simulink model "Buck_Converter_with_3ph_Full_Bridge_Rectifier_v2"  (R2022b)
settings: Solver=VariableStepAuto  StartTime=0.0  StopTime=3  RelTol=1e-3
libraries: spsDiodeLib x7, spsRMSLib x4, spsCurrentMeasurementLib x3, spsSeriesRLCBranchLib x3, spsVoltageMeasurementLib x2, slpidlib x1, simulink x1, spsDCMachineLib x1, spsDCVoltageSourceLib x1, spsGroundLib x1, spsIGBTDiodeLib x1, spsPower3phInstantaneousLib x1
settings Model: Creator=meteh  LastModifiedBy=meteh
settings SolverCC: ZeroCrossAlgorithm=Adaptive
settings DebuggingCC: IgnoredZcDiagnostic=none

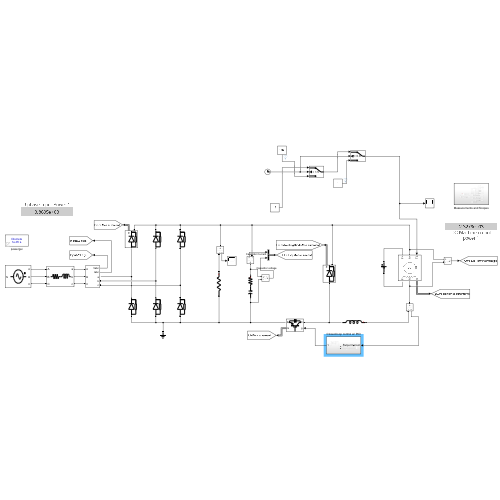
[thumbnail: Simulink's stored preview of the top-level diagram]
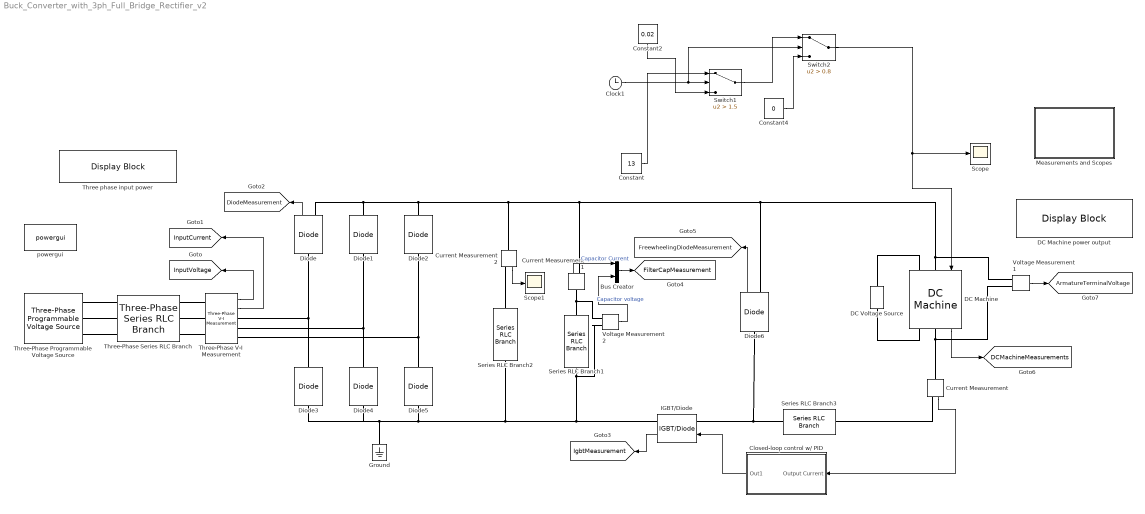
== system Buck_Converter_with_3ph_Full_Bridge_Rectifier_v2 ==
  Bus Creator : BusCreator  Inputs=2
  Clock1 : Clock
  Closed-loop control w/ PID : Subsystem
  Constant : Constant  Value=13
  Constant2 : Constant  Value=0.02
  Constant4 : Constant  Value=0
  Current Measurement : spsCurrentMeasurementLib/Current Measurement  PhasorSimulation=off  OutputType=Complex  PSBequivalent=0
  Current Measurement1 : spsCurrentMeasurementLib/Current Measurement  PhasorSimulation=off  OutputType=Complex  PSBequivalent=0
  Current Measurement2 : spsCurrentMeasurementLib/Current Measurement  PhasorSimulation=off  OutputType=Complex  PSBequivalent=0
  DC Machine : spsDCMachineLib/DC Machine  PresetModel=No  MechanicalLoad=Torque TL  FieldType=Wound  ShowDetailedParameters=on  MeasurementBus=off  RLa="[ 0.8  0.0125]"  RLf="[ 210  23]"  Laf=1  MachineConstant=Torque constant (N.m/A)  Ke=1.8  Kt=1.8  J=0.001  Bm=0.001  Tf=0.001  w0=0  Ifinit=0  TsPowergui=0  TsBlock=-1
  DC Machine power output : DisplayBlock  LabelPosition=Bottom  Transparency=1
  DC Voltage Source : spsDCVoltageSourceLib/DC Voltage Source  Amplitude=200  Measurements=None
  Diode : spsDiodeLib/Diode  Ron=0.001  Lon=0  Vf=0.8  IC=0  UseSnubber=0  Rs=500  Cs=250e-9  Measurements=on
  Diode{1..5} (5 alike) : spsDiodeLib/Diode  Ron=0.001  Lon=0  Vf=0.8  IC=0  UseSnubber=0  Rs=500  Cs=250e-9  Measurements=off
  Diode6 : spsDiodeLib/Diode  Ron=0.001  Lon=0  Vf=0.8  IC=0  UseSnubber=0  Rs=120  Cs=250e-9  Measurements=on
  Ground : spsGroundLib/Ground  LConnTagsString=a
  IGBT/Diode : spsIGBTDiodeLib/IGBT//Diode  Ron=1e-2  Rs=120  Cs=250e-9  Measurements=on
  Measurements and Scopes : Subsystem
  Scope : Scope
  Scope1 : Scope
  Series RLC Branch1 : spsSeriesRLCBranchLib/Series RLC Branch  LConnTagsString=__new0  RConnTagsString=__new0  BranchType=RC  Resistance=0.01  Inductance=12.5e-3  SetiL0=off  InitialCurrent=0  Capacitance=940e-6  Setx0=off  InitialVoltage=0  Measurements=None
  Series RLC Branch2 : spsSeriesRLCBranchLib/Series RLC Branch  LConnTagsString=__new0  RConnTagsString=__new0  BranchType=R  Resistance=5.6e3  Inductance=12.5e-3  SetiL0=off  InitialCurrent=0  Capacitance=940e-6  Setx0=off  InitialVoltage=0  Measurements=None
  Series RLC Branch3 : spsSeriesRLCBranchLib/Series RLC Branch  LConnTagsString=__new0  RConnTagsString=__new0  BranchType=L  Resistance=0.01  Inductance=10e-9  SetiL0=off  InitialCurrent=0  Capacitance=940e-6  Setx0=off  InitialVoltage=0  Measurements=None
  Switch1 : Switch  Criteria=u2 > Threshold  Threshold=1.5  SaturateOnIntegerOverflow=off  InputSameDT=off
  Switch2 : Switch  Criteria=u2 > Threshold  Threshold=0.8  SaturateOnIntegerOverflow=off  InputSameDT=off
  Three phase input power : DisplayBlock  Description=Three phase input power  Transparency=1  Layout=Fill available space
  Three-Phase Programmable Voltage Source : spsThreePhaseProgrammableVoltageSourceLib/Three-Phase Programmable Voltage Source  PositiveSequence="[133  0 50]"  VariationEntity=Amplitude  VariationType=Table of time-amplitude pairs  VariationTypeAlt=Step  VariationStep=0.5  VariationRate=10  VariationMagnitude=0.3  VariationFrequency=2  VariationTiming=[1 2]  VariationPhaseA=off  Amplitudes=[0 0.25 0.5 0.75 1.0]  TimeValues=[0 0.2 0.4 0.6 0.8]  HarmonicGeneration=off  HarmonicA=[3 0.2 -25 0]  HarmonicB=[2 0.15 35 2]  Timing="[0.05  3]"  BusType=swing  Pref=0  Qref=0  Qmin=-inf  Qmax=inf
  Three-Phase Series RLC Branch : spsThreePhaseSeriesRLCBranchLib/Three-Phase Series RLC Branch  LConnTagsString=A|B|C  RConnTagsString=A|B|C  BranchType=RL  Resistance=1e-3  Inductance=2e-3  Capacitance=1e-6  Measurements=None
  Three-Phase V-I Measurement : spsThreePhaseVIMeasurementLib/Three-Phase V-I Measurement  VoltageMeasurement=phase-to-ground  SetLabelV=off  LabelV=Vabc  Vpu=off  VpuLL=off  CurrentMeasurement=yes  SetLabelI=off  LabelI=Iabc  Ipu=off  Pbase=100e6  Vbase=500e3  OutputType=Complex  PhasorSimulation=off  PSBequivalent=0
  Voltage Measurement1 : spsVoltageMeasurementLib/Voltage Measurement  PhasorSimulation=off  OutputType=Complex  PSBequivalent=0
  Voltage Measurement2 : spsVoltageMeasurementLib/Voltage Measurement  PhasorSimulation=off  OutputType=Complex  PSBequivalent=0
  powergui : spspowerguiLib/powergui  Priority=1  SimulationMode=Discrete  SampleTime=1e-5  frequency=60  Iterations=50  frequencyindice=0  Pbase=100e6  ErrMax=1e-4  UnitsV=kV  UnitsW=MW  buscounter=0  FunctionMessages=off  echomessages=off  EnableUseOfTLC=off  CurrentSourceSwitches=on  DisableSnubberDevices=off  DisableRonSwitches=off  DisableVfSwitches=off  DisplayEquations=off  AutomaticDiscreteSolvers=off  SolverType=Tustin/Backward Euler (TBE)  Interpol=off  ExternalGateDelay=off  methode=off  Ts=100  x0status=zero  SPID=on  SwTol=0  HookPort=off  NonlinearTolerance=1e-4  nMaxIteration=100  ContinueOnMaxIteration=off  RestoreLinks=warning  ResistiveCurrentMeasurement=off  Frange=[0:2:500]  Ylog=off  Xlog=on  ShowGrid=off  save=off  variable=ZData  structure=0  ZoomFFT=off  StartTime=0.0  cycles=1  DisplayStyle=1  fundamental=60  FreqAxis=off  MaxFrequency=1000  frequencyindicesteady=1  RmsSteady=1  display=off
  tag scope: ArmatureTerminalVoltage=global, DCMachineMeasurements=global, DiodeMeasurement=global, FilterCapMeasurement=global, FreewheelingDiodeMeasurement=global, IgbtMeasurement=global, InputCurrent=global, InputVoltage=global
  wires:
  Switch2/1 -> Scope/1, DC Machine/1
  Three-Phase V-I Measurement/2 -> [InputCurrent]
  Three-Phase V-I Measurement/1 -> [InputVoltage]
  Diode6/1 -> [FreewheelingDiodeMeasurement]
  Current Measurement1/1 -> Bus Creator/1  "Capacitor Current"
  Voltage Measurement2/1 -> Bus Creator/2  "Capacitor voltage"
  Bus Creator/1 -> [FilterCapMeasurement]
  DC Machine/1 -> [DCMachineMeasurements]
  Voltage Measurement1/1 -> [ArmatureTerminalVoltage]
  Diode/1 -> [DiodeMeasurement]
  IGBT/Diode/1 -> [IgbtMeasurement]
  Closed-loop control w/ PID/1(Out1) -> IGBT/Diode/1
  Current Measurement/1 -> Closed-loop control w/ PID/1(Output Current)
  Current Measurement2/1 -> Scope1/1
  Switch1/1 -> Switch2/1
  Constant4/1 -> Switch2/3
  Constant2/1 -> Switch1/3
  Constant/1 -> Switch1/1
  Clock1/1 -> Switch2/2, Switch1/2
  connections:
  Diode3/RConn1 -- Three-Phase V-I Measurement/RConn1 -- Diode/LConn1
  Diode4/RConn1 -- Three-Phase V-I Measurement/RConn2 -- Diode1/LConn1
  Diode5/RConn1 -- Diode2/LConn1 -- Three-Phase V-I Measurement/RConn3
  Series RLC Branch1/RConn1 -- IGBT/Diode/RConn1 -- Series RLC Branch2/RConn1 -- Ground/LConn1 -- Diode3/LConn1 -- Diode4/LConn1 -- Diode5/LConn1 -- Voltage Measurement2/LConn2
  DC Voltage Source/RConn1 -- DC Machine/LConn2
  DC Machine/RConn2 -- DC Voltage Source/LConn1
  Current Measurement1/RConn1 -- Voltage Measurement1/LConn1 -- DC Machine/LConn1 -- Diode6/RConn1 -- Current Measurement2/LConn1 -- Diode/RConn1 -- Diode1/RConn1 -- Diode2/RConn1
  Current Measurement1/LConn1 -- Series RLC Branch1/LConn1 -- Voltage Measurement2/LConn1
  Current Measurement/RConn1 -- Series RLC Branch3/LConn1
  DC Machine/RConn1 -- Current Measurement/LConn1 -- Voltage Measurement1/LConn2
  Series RLC Branch3/RConn1 -- Diode6/LConn1 -- IGBT/Diode/LConn1
  Series RLC Branch2/LConn1 -- Current Measurement2/RConn1
  Three-Phase Programmable Voltage Source/RConn3 -- Three-Phase Series RLC Branch/LConn3
  Three-Phase Programmable Voltage Source/RConn2 -- Three-Phase Series RLC Branch/LConn2
  Three-Phase Programmable Voltage Source/RConn1 -- Three-Phase Series RLC Branch/LConn1
  Three-Phase Series RLC Branch/RConn1 -- Three-Phase V-I Measurement/LConn1
  Three-Phase Series RLC Branch/RConn2 -- Three-Phase V-I Measurement/LConn2
  Three-Phase Series RLC Branch/RConn3 -- Three-Phase V-I Measurement/LConn3

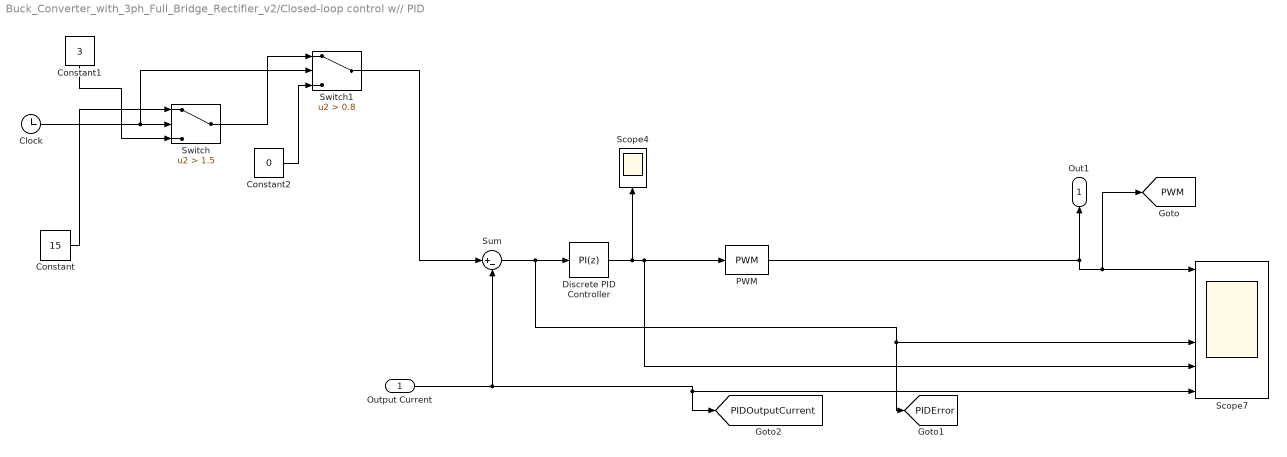
== system Buck_Converter_with_3ph_Full_Bridge_Rectifier_v2/Closed-loop control w// PID ==
  Output Current : Inport
  Clock : Clock
  Constant : Constant  Value=15
  Constant1 : Constant  Value=3
  Constant2 : Constant  Value=0
  Discrete PID Controller : slpidlib/PID Controller  Controller=PI  Form=Parallel  TimeDomain=Discrete-time  UseExternalTs=off  SampleTime=1/25000  IntegratorMethod=Forward Euler  FilterMethod=Forward Euler  ControllerParametersSource=internal  P=80  I=10  UseKiTs=off  D=0  N=100  UseFilter=on  TunerSelectOption=Transfer Function Based (PID Tuner App)  InitialConditionSource=internal  InitialConditionForIntegrator=0  InitialConditionForFilter=0  DifferentiatorICPrevScaledInput=0  ExternalReset=none  TrackingMode=off  Kt=1  LimitOutput=on  SatLimitsSource=internal  UpperSaturationLimit=1  LowerSaturationLimit=0  LinearizeAsGain=off  AntiWindupMode=none  Kb=1  LimitIntegrator=off  UpperIntegratorSaturationLimit=inf  LowerIntegratorSaturationLimit=-inf  POutMin=[]  POutMax=[]  IOutMin=[]  IOutMax=[]  DOutMin=[]  DOutMax=[]  NOutMin=[]  NOutMax=[]  SumOutMin=[]  SumOutMax=[]  SaturationOutMin=[]  SaturationOutMax=[]  PParamMin=[]  PParamMax=[]  IParamMin=[]  IParamMax=[]  DParamMin=[]  DParamMax=[]  NParamMin=[]  NParamMax=[]  KbParamMin=[]  KbParamMax=[]  KtParamMin=[]  KtParamMax=[]  KbOutMin=[]  KbOutMax=[]  KtOutMin=[]  KtOutMax=[]  IntegratorOutMin=[]  IntegratorOutMax=[]  FilterOutMin=[]  FilterOutMax=[]  SumI1OutMin=[]  SumI1OutMax=[]  SumI2OutMin=[]  SumI2OutMax=[]  SumI3OutMin=[]  SumI3OutMax=[]  SumI4OutMin=[]  SumI4OutMax=[]  SumDOutMin=[]  SumDOutMax=[]  DifferentiatorOutMin=[]  DifferentiatorOutMax=[]  FilterDiffOutCoefMin=[]  FilterDiffOutCoefMax=[]  ReciprocalOutMin=[]  ReciprocalOutMax=[]  SumDenOutMin=[]  SumDenOutMax=[]  SumNumOutMin=[]  SumNumOutMax=[]  DivideOutMin=[]  DivideOutMax=[]  UdiffTsProdOutMin=[]  UdiffTsProdOutMax=[]  NTsProdOutMin=[]  NTsProdOutMax=[]  UintegralTsProdOutMin=[]  UintegralTsProdOutMax=[]  UngainTsProdOutMin=[]  UngainTsProdOutMax=[]  ClampingZeroOutDataTypeStr=Inherit: Inherit via back propagation  ClampingZeroOutMin=[]  ClampingZeroOutMax=[]  FilterDenConstantOutDataTypeStr=Inherit: Inherit via back propagation  FilterDenConstantOutMin=[]  FilterDenConstantOutMax=[]  PCopyOutDataTypeStr=Inherit: Inherit via back propagation  PCopyOutMin=[]  PCopyOutMax=[]  NCopyOutDataTypeStr=Inherit: Inherit via back propagation  NCopyOutMin=[]  NCopyOutMax=[]  IntegratorContinuousStateAttributes=''  IntegratorStateMustResolveToSignalObject=off  IntegratorRTWStateStorageClass=Auto  FilterContinuousStateAttributes=''  FilterStateMustResolveToSignalObject=off  FilterRTWStateStorageClass=Auto  ParallelPVariant=InternalParameters  IdealPVariant=Disabled  IVariant=InternalParameters  DVariant=Disabled  IntegratorVariant=Discrete  SatVariant=Enabled  AWVariant=Passthrough  PCopyVariant=Disabled  TRVariant=Disabled  FdbkBlocksVariant=Forward  IdealPFdbkVariant=Disabled  SatFdbkVariant=Disabled  DerivativeFilterVariant=Disabled  NVariant=Disabled  NCopyVariant=Disabled_SignalSpec  FilterICVariant=Disabled  IntegratorICVariant=InternalICs  ExternalResetVariant=Disabled  TRSumVariant=Passthrough  SumFdbkVariant=Disabled  SumVariant=Sum_PI  TsampFilterVariant=InternalTs  TsampNgainVariant=Passthrough  TsampIntegralVariant=Passthrough  ExternalSaturationOutDataTypeStr=Inherit: Same as second input
      settings: LibrarySourceBlock=simulink/Discrete/Discrete PID Controller
  PWM : simulink/Discontinuities/PWM  DisableCoverage=on  Period=1/25000  InitialDelay=0  DisallowZeroDutyCycle=off  RunAtFixedTimeIntervals=on  SampleTime=5e-6
  Scope4 : Scope
  Scope7 : Scope  NumInputPorts=6
  Sum : Sum  Inputs=|+-
  Switch : Switch  Criteria=u2 > Threshold  Threshold=1.5  SaturateOnIntegerOverflow=off  InputSameDT=off
  Switch1 : Switch  Criteria=u2 > Threshold  Threshold=0.8  SaturateOnIntegerOverflow=off  InputSameDT=off
  Out1 : Outport
  tag scope: PIDError=global, PIDOutputCurrent=global, PWM=global
  wires:
  Sum/1 -> Discrete PID Controller/1, [PIDError], Scope7/4
  Discrete PID Controller/1 -> PWM/1, Scope7/5, Scope4/1
  Output Current/1 -> Sum/2, Scope7/6, [PIDOutputCurrent]
  PWM/1 -> [PWM], Scope7/1, Out1/1
  Constant/1 -> Switch/1
  Constant1/1 -> Switch/3
  Clock/1 -> Switch1/2, Switch/2
  Switch1/1 -> Sum/1
  Switch/1 -> Switch1/1
  Constant2/1 -> Switch1/3

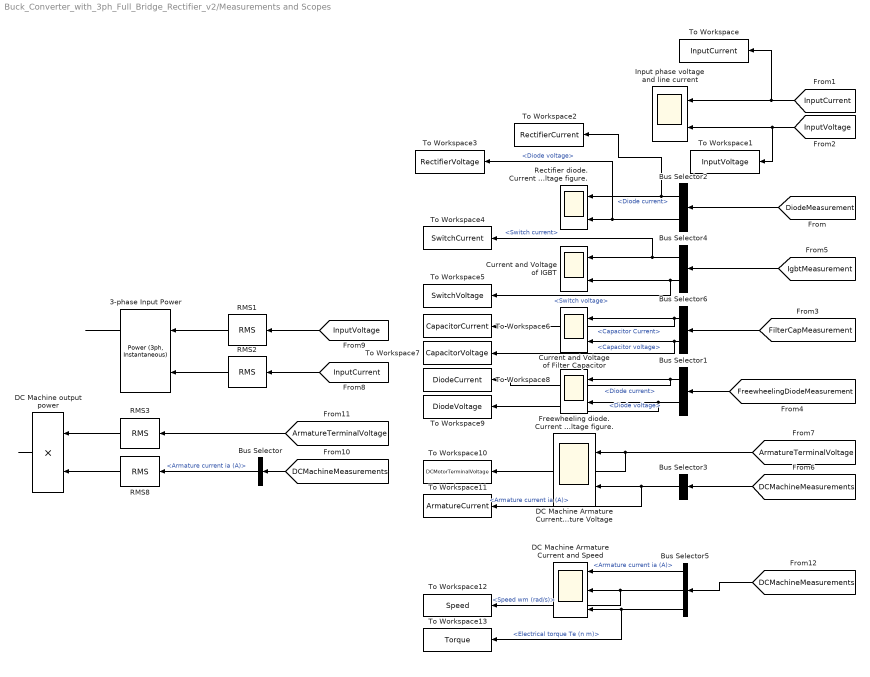
== system Buck_Converter_with_3ph_Full_Bridge_Rectifier_v2/Measurements and Scopes ==
  3-phase Input Power : spsPower3phInstantaneousLib/Power (3ph, Instantaneous)
  Bus Selector : BusSelector  OutputSignals=Armature current ia (A)
  Bus Selector1 : BusSelector  OutputSignals=Diode current,Diode voltage
  Bus Selector2 : BusSelector  OutputSignals=Diode current,Diode voltage
  Bus Selector3 : BusSelector  OutputSignals=Armature current ia (A)
  Bus Selector4 : BusSelector  OutputSignals=Switch current,Switch voltage
  Bus Selector5 : BusSelector  OutputSignals=Armature current ia (A),Speed wm (rad/s),Electrical torque Te (n m)
  Bus Selector6 : BusSelector  OutputSignals=Capacitor Current,Capacitor voltage
  Current and Voltage of Filter Capacitor : Scope  NumInputPorts=2
  Current and Voltage of IGBT : Scope  NumInputPorts=2
  DC Machine Armature Current and Armature Voltage : Scope  NumInputPorts=2
  DC Machine Armature Current and Speed : Scope  NumInputPorts=3
  DC Machine output power : Product
  Freewheeling diode. Current and Voltage figure. : Scope  NumInputPorts=2
  Input phase voltage and line current : Scope  NumInputPorts=2
  RMS1 : spsRMSLib/RMS  TrueRMS=on  Freq=50  RMSInit=0  Ts=0
  RMS2 : spsRMSLib/RMS  TrueRMS=on  Freq=50  RMSInit=0  Ts=0
  RMS3 : spsRMSLib/RMS  TrueRMS=on  Freq=50  RMSInit=0  Ts=0
  RMS8 : spsRMSLib/RMS  TrueRMS=on  Freq=60  RMSInit=0  Ts=0
  Rectifier diode. Current and voltage figure. : Scope  NumInputPorts=2
  To Workspace : ToWorkspace  VariableName=InputCurrent  SaveFormat=Timeseries  SampleTime=-1
  To Workspace1 : ToWorkspace  VariableName=InputVoltage  SaveFormat=Timeseries  SampleTime=-1
  To Workspace10 : ToWorkspace  VariableName=DCMotorTerminalVoltage  SaveFormat=Timeseries  SampleTime=-1
  To Workspace11 : ToWorkspace  VariableName=ArmatureCurrent  SaveFormat=Timeseries  SampleTime=-1
  To Workspace12 : ToWorkspace  VariableName=Speed  SaveFormat=Timeseries  SampleTime=-1
  To Workspace13 : ToWorkspace  VariableName=Torque  SaveFormat=Timeseries  SampleTime=-1
  To Workspace2 : ToWorkspace  VariableName=RectifierCurrent  SaveFormat=Timeseries  SampleTime=-1
  To Workspace3 : ToWorkspace  VariableName=RectifierVoltage  SaveFormat=Timeseries  SampleTime=-1
  To Workspace4 : ToWorkspace  VariableName=SwitchCurrent  SaveFormat=Timeseries  SampleTime=-1
  To Workspace5 : ToWorkspace  VariableName=SwitchVoltage  SaveFormat=Timeseries  SampleTime=-1
  To Workspace6 : ToWorkspace  VariableName=CapacitorCurrent  SaveFormat=Timeseries  SampleTime=-1
  To Workspace7 : ToWorkspace  VariableName=CapacitorVoltage  SaveFormat=Timeseries  SampleTime=-1
  To Workspace8 : ToWorkspace  VariableName=DiodeCurrent  SaveFormat=Timeseries  SampleTime=-1
  To Workspace9 : ToWorkspace  VariableName=DiodeVoltage  SaveFormat=Timeseries  SampleTime=-1
  wires:
  Bus Selector/1 -> RMS8/1  "<Armature current ia (A)>"
  [FreewheelingDiodeMeasurement] -> Bus Selector1/1
  Bus Selector1/1 -> Freewheeling diode. Current and Voltage figure./1, To Workspace8/1  "<Diode current>"
  Bus Selector1/2 -> Freewheeling diode. Current and Voltage figure./2, To Workspace9/1  "<Diode voltage>"
  [DiodeMeasurement] -> Bus Selector2/1
  Bus Selector2/1 -> Rectifier diode. Current and voltage figure./1, To Workspace2/1  "<Diode current>"
  Bus Selector2/2 -> Rectifier diode. Current and voltage figure./2, To Workspace3/1  "<Diode voltage>"
  [ArmatureTerminalVoltage] -> To Workspace10/1, DC Machine Armature Current and Armature Voltage/1
  [DCMachineMeasurements] -> Bus Selector3/1
  Bus Selector3/1 -> To Workspace11/1, DC Machine Armature Current and Armature Voltage/2  "<Armature current ia (A)>"
  [IgbtMeasurement] -> Bus Selector4/1
  Bus Selector4/1 -> Current and Voltage of IGBT/1, To Workspace4/1  "<Switch current>"
  Bus Selector4/2 -> Current and Voltage of IGBT/2, To Workspace5/1  "<Switch voltage>"
  [DCMachineMeasurements] -> Bus Selector/1
  [DCMachineMeasurements] -> Bus Selector5/1
  Bus Selector5/1 -> DC Machine Armature Current and Speed/1  "<Armature current ia (A)>"
  Bus Selector5/2 -> To Workspace12/1, DC Machine Armature Current and Speed/2  "<Speed wm (rad/s)>"
  Bus Selector6/2 -> Current and Voltage of Filter Capacitor/2, To Workspace7/1  "<Capacitor voltage>"
  Bus Selector6/1 -> Current and Voltage of Filter Capacitor/1, To Workspace6/1  "<Capacitor Current>"
  [FilterCapMeasurement] -> Bus Selector6/1
  [InputCurrent] -> To Workspace/1, Input phase voltage and line current/1
  [InputVoltage] -> To Workspace1/1, Input phase voltage and line current/2
  3-phase Input Power/1 -> ?
  [ArmatureTerminalVoltage] -> RMS3/1
  [InputVoltage] -> RMS1/1
  [InputCurrent] -> RMS2/1
  RMS3/1 -> DC Machine output power/1
  RMS1/1 -> 3-phase Input Power/1
  RMS2/1 -> 3-phase Input Power/2
  RMS8/1 -> DC Machine output power/2
  DC Machine output power/1 -> ?
  Bus Selector5/3 -> To Workspace13/1, DC Machine Armature Current and Speed/3  "<Electrical torque Te (n m)>"
